simulink model "pid_controller"  (R2020a)
settings: Solver=VariableStepAuto  StartTime=0.0  StopTime=10.0  RelTol=1e-3
values from neighbouring files (symbols this model uses):
  kd = 346    [week2prob3.mat]
  ki = 76    [week2prob3.mat]
  kp = 1000    [week2prob3.mat]
settings Model: Creator=Admin  LastModifiedBy=Admin
settings DataIOCC: SaveOutput=off  SaveTime=off

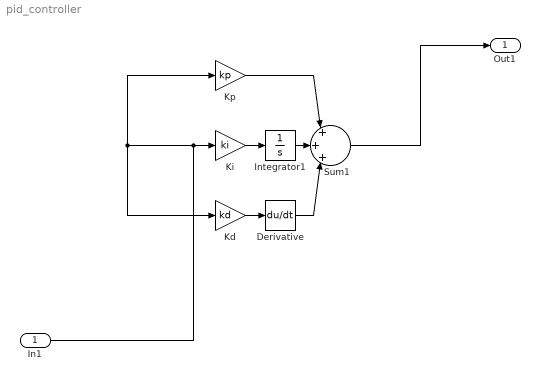
== system pid_controller ==
  In1 : Inport  OutDataTypeStr=double  PortDimensions=1  SampleTime=0
  Derivative : Derivative
  Integrator1 : Integrator
  Kd : Gain  Gain=kd
  Ki : Gain  Gain=ki
  Kp : Gain  Gain=kp
  Sum1 : Sum  Inputs=|+|+|+|
  Out1 : Outport  OutDataTypeStr=double  PortDimensions=1  SampleTime=0
  wires:
  Ki/1 -> Integrator1/1
  In1/1 -> Ki/1, Kd/1, Kp/1
  Integrator1/1 -> Sum1/2
  Kd/1 -> Derivative/1
  Kp/1 -> Sum1/1
  Derivative/1 -> Sum1/3
  Sum1/1 -> Out1/1
